simulink library "genericAgentLib"  (R2019a)
settings: Solver=VariableStepAuto  StartTime=0.0  StopTime=10.0  RelTol=1e-3
undefined symbols (not defined in the file or in its folder): Objects
libraries: $bdroot x1
settings Model: Creator=swami  LastModifiedBy=akshay

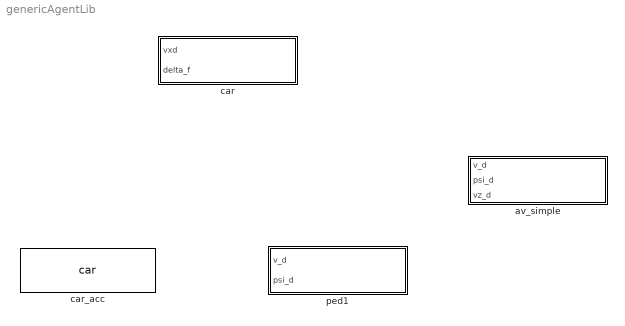
== system genericAgentLib ==
  av_simple : Subsystem  mask{obj=Objects{6}}
      mask prompts: obj "object"
      mask init:
      | set_param([gcb,'/ToWS'],'VariableName',obj.NameStrh)
  car : Subsystem  mask{obj=Objects{1}}
      mask prompts: obj "object"
      mask init:
      | set_param([gcb,'/ToWS'],'VariableName',obj.NameStrh)
  car_acc : $bdroot/car  obj=Objects{1}
  ped1 : Subsystem  mask{obj=Objects{3}}
      mask prompts: obj "object"
      mask init:
      | set_param([gcb,'/ToWS'],'VariableName',obj.NameStrh)

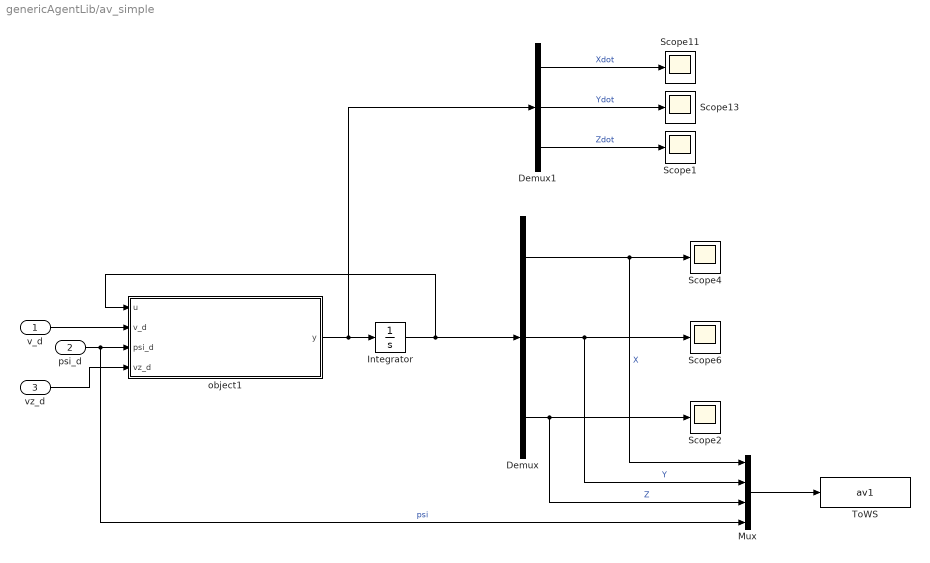
== system genericAgentLib/av_simple ==
  v_d : Inport
  psi_d : Inport  Port=2
  vz_d : Inport  Port=3
  Demux : Demux  Outputs=3
  Demux1 : Demux  Outputs=3
  Integrator : Integrator  InitialCondition=obj.init
  Mux : Mux
  Scope{1..2,4,6,11,13} (6 alike) : Scope
  ToWS : ToWorkspace  VariableName=av1  SaveFormat=Timeseries  SampleTime=-1
  object1 : MATLAB Function  TreatAsAtomicUnit=on
  wires:
  Demux/2 -> Mux/2, Scope6/1  "Y"
  Demux/1 -> Mux/1, Scope4/1  "X"
  psi_d/1 -> Mux/4, object1/3(psi_d)  "psi"
  v_d/1 -> object1/2(v_d)
  Mux/1 -> ToWS/1
  object1/1(y) -> Integrator/1, Demux1/1
  Demux1/1 -> Scope11/1  "Xdot"
  Demux1/2 -> Scope13/1  "Ydot"
  Integrator/1 -> object1/1(u), Demux/1
  vz_d/1 -> object1/4(vz_d)
  Demux1/3 -> Scope1/1  "Zdot"
  Demux/3 -> Mux/3, Scope2/1  "Z"

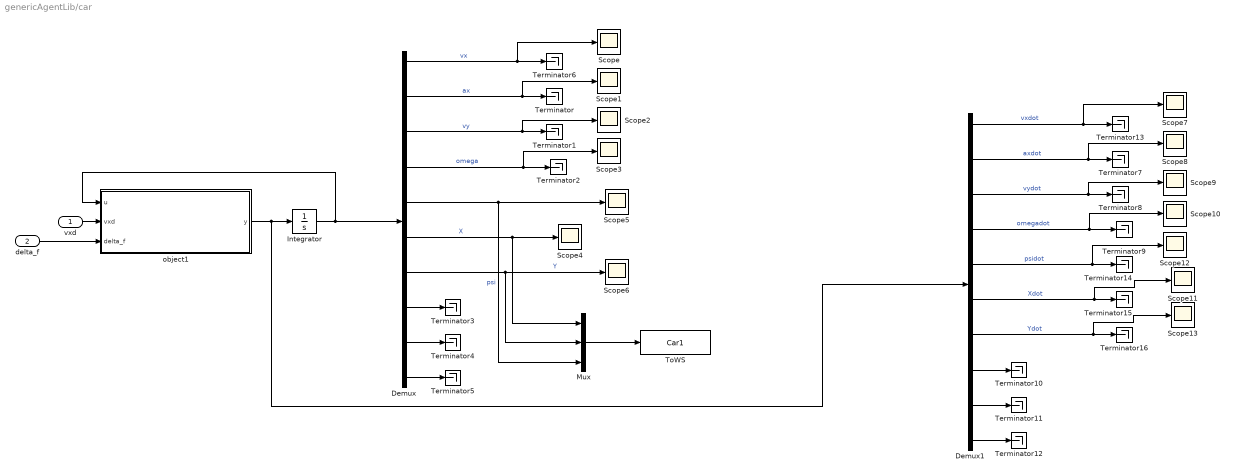
== system genericAgentLib/car ==
  "vxd " : Inport
  delta_f : Inport  Port=2
  Demux : Demux  Outputs=10
  Demux1 : Demux  Outputs=10
  Integrator : Integrator  InitialCondition=obj.init
  Mux : Mux  Inputs=3
  Scope{,1..13} (14 alike) : Scope
  Terminator{,1..16} (17 alike) : Terminator
  ToWS : ToWorkspace  VariableName=Car1  SaveFormat=Timeseries  SampleTime=-1
  object1 : MATLAB Function  TreatAsAtomicUnit=on
  wires:
  Integrator/1 -> Demux/1, object1/1(u)
  delta_f/1 -> object1/3(delta_f)
  Demux/1 -> Scope/1, Terminator6/1  "vx"
  Demux/2 -> Scope1/1, Terminator/1  "ax"
  Demux/3 -> Scope2/1, Terminator1/1  "vy"
  Demux/4 -> Scope3/1, Terminator2/1  "omega"
  Demux/5 -> Mux/3, Scope5/1  "psi"
  Demux/6 -> Mux/1, Scope4/1  "X"
  Demux/7 -> Mux/2, Scope6/1  "Y"
  Demux/8 -> Terminator3/1
  Demux/9 -> Terminator4/1
  Demux/10 -> Terminator5/1
  Demux1/10 -> Terminator12/1
  Demux1/9 -> Terminator11/1
  Demux1/8 -> Terminator10/1
  Demux1/7 -> Terminator16/1, Scope13/1  "Ydot"
  Demux1/6 -> Terminator15/1, Scope11/1  "Xdot"
  Demux1/5 -> Terminator14/1, Scope12/1  "psidot"
  Demux1/4 -> Terminator9/1, Scope10/1  "omegadot"
  Demux1/3 -> Terminator8/1, Scope9/1  "vydot"
  Demux1/2 -> Terminator7/1, Scope8/1  "axdot"
  Demux1/1 -> Terminator13/1, Scope7/1  "vxdot"
  object1/1(y) -> Demux1/1, Integrator/1
  Mux/1 -> ToWS/1
  "vxd "/1 -> object1/2(vxd)

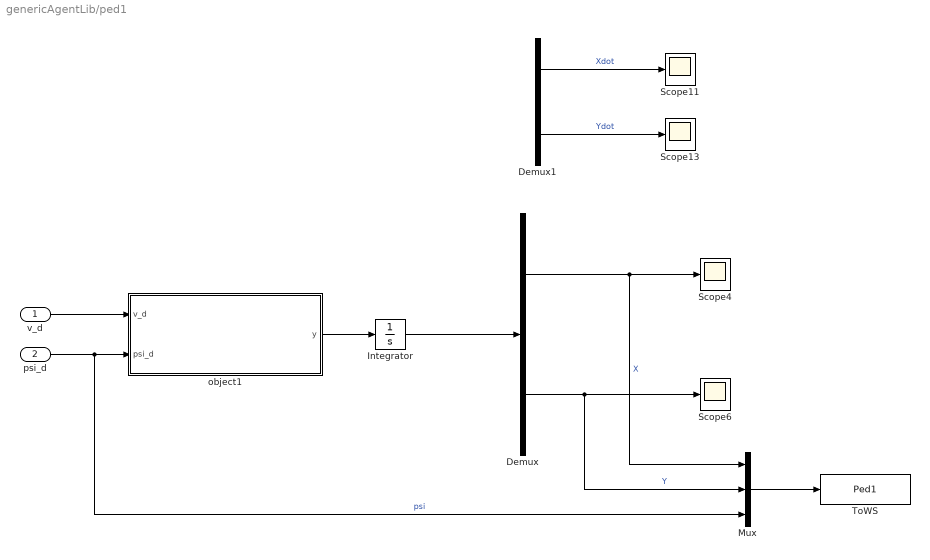
== system genericAgentLib/ped1 ==
  v_d : Inport
  psi_d : Inport  Port=2
  Demux : Demux  Outputs=2
  Demux1 : Demux  Outputs=2
  Integrator : Integrator  InitialCondition=obj.init
  Mux : Mux  Inputs=3
  Scope{4,6,11,13} (4 alike) : Scope
  ToWS : ToWorkspace  VariableName=Ped1  SaveFormat=Timeseries  SampleTime=-1
  object1 : MATLAB Function  TreatAsAtomicUnit=on
  wires:
  object1/1(y) -> Integrator/1
  Demux/2 -> Scope6/1, Mux/2  "Y"
  Demux/1 -> Scope4/1, Mux/1  "X"
  psi_d/1 -> object1/2(psi_d), Mux/3  "psi"
  Mux/1 -> ToWS/1
  Demux1/1 -> Scope11/1  "Xdot"
  Demux1/2 -> Scope13/1  "Ydot"
  Integrator/1 -> Demux/1
  v_d/1 -> object1/1(v_d)

== matlab function genericAgentLib/ped1/object1 ==
  data: v_d input; psi_d input; y output size=2; obj parameter
function y = pedObject(v_d, psi_d, obj)

Xdot = v_d * cos(psi_d);
Ydot = v_d * sin(psi_d);
y = [Xdot, Ydot]';
end

function y = TF(psi)
y = [cos(psi), sin(psi); -sin(psi), cos(psi)];
end

== matlab function genericAgentLib/car/object1 ==
  data: u input size=10; vxd input size=1; delta_f input size=1; y output size=10; obj parameter
function y = fcn(u,vxd, delta_f, obj)

vx = u(1);
ax = u(2);
vy = u(3);
omega = u(4);
psi = u(5);
X = u(6);
Y = u(7);

if abs(vx)> obj.vx_threshold1
    alpha_f = delta_f * pi/180 - (vy + omega * obj.lf) / vx;
    alpha_r = - (vy - omega * obj.lr) / vx;
else
    alpha_f = 0;
    alpha_r = 0;
end

Fx = obj.m * ax;
Fyf = min(obj.Fyfmax,obj.Calpha_f * alpha_f);
Fyr = min(obj.Fyrmax, obj.Calpha_r * alpha_r);
Fy = Fyf + Fyr;

M  = Fyf * obj.lf - Fyr * obj.lr;

omegadot = M / obj.I;
%        vxdot = Fx / obj.m + omega * vy;
vxdot = ax;
axdot = - 2 * obj.longctl.psi * obj.longctl.w* ax - (obj.longctl.w)^2 * (vx - vxd);
vydot = Fy / obj.m - omega * vx;
psidot = omega;
t1 = TF(psi) * [vx;vy];
Xdot = t1(1);
Ydot = t1(2);
y = [vxdot, axdot, vydot, omegadot, psidot, Xdot, Ydot, 0 0 0]';
end

function y = TF(psi)
y = [cos(psi), sin(psi); -sin(psi), cos(psi)];
end

== matlab function genericAgentLib/av_simple/object1 ==
  data: u input; v_d input; psi_d input; vz_d input; y output size=3; obj parameter
function y = fcn(u, v_d, psi_d, vz_d, obj)

Z = u(3);
Xdot = v_d * cos(psi_d);
Ydot = v_d * sin(psi_d);
if Z <= 0 && vz_d < 0
   Zdot = 0;
else
   Zdot = vz_d;
end
y = [Xdot, Ydot, Zdot]';
end

function y = TF(psi)
y = [cos(psi), sin(psi); -sin(psi), cos(psi)];
end
